simulink model "temperatureSource"  (R2016b)
settings: Solver=VariableStepAuto  StartTime=0.0  StopTime=10.0  RelTol=1e-3
libraries: fl_lib x4, nesl_utility x3
settings Model: Creator=Taeke  LastModifiedBy=Taeke

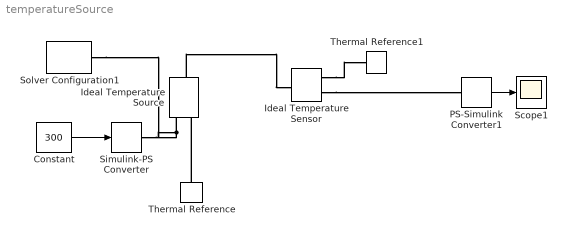
== system temperatureSource ==
  Constant : Constant  Value=300
  Ideal Temperature Sensor : fl_lib/Thermal/Thermal Sensors/Ideal Temperature Sensor
  Ideal Temperature Source : fl_lib/Thermal/Thermal Sources/Ideal Temperature Source
  PS-Simulink Converter1 : nesl_utility/PS-Simulink Converter  PhysicalDomain=network_engine_domain  SubClassName=ps_output  LeftPortType=input  RightPortType=output  PseudoPeriodic=off  Frequencies=[]  Unit=1  AffineConversion=off
  Scope1 : Scope
  Simulink-PS Converter : nesl_utility/Simulink-PS Converter  PhysicalDomain=network_engine_domain  SubClassName=ps_input  LeftPortType=input  RightPortType=output  PseudoPeriodic=off  Frequencies=[]  NoiseDistribution=none  NoiseParameters=[]  Unit=1  AffineConversion=off  InputFiltering=off  SimscapeFilterOrder=1  InputFilterTimeConstant=0.001  UdotUserProvided=1
  Solver Configuration1 : nesl_utility/Solver Configuration  PhysicalDomain=network_engine_domain  SubClassName=solver  LeftPortType=input  RightPortType=generic  Accelerate=off  Tones=[]  Harmonics=[]  SimulateNoise=off  Profile=off  UseLocalSampling=off  EnableSwitchedLinearOptims=on  FrequencyDomain=off  UseCCode=off  RelTol=0.001  AbsTol=1e-06  MinStep=1e-09  ToWorkspace=off  RevertToSquareIcSolve=off  NumHomotopyIterations=100  PhasorMode=off  PhasorModeNumHarmonics=1  OverrideAbsTol=off  DoDC=off  ResidualTolerance=1e-09  UseLocalSolver=off  LocalSolverChoice=NE_BACKWARD_EULER_ADVANCER  LocalSolverSampleTime=0.001  DoFixedCost=off  MaxNonlinIter=3  MaxModeIter=2  LinearAlgebra=Sparse  DelaysMemoryBudget=1024  AutomaticFiltering=on  FilteringTimeConstant=0.001
  Thermal Reference : fl_lib/Thermal/Thermal Elements/Thermal Reference
  Thermal Reference1 : fl_lib/Thermal/Thermal Elements/Thermal Reference
  wires:
  Constant/1 -> Simulink-PS Converter/1
  PS-Simulink Converter1/1 -> Scope1/1
  connections:
  Ideal Temperature Source/RConn1 -- Simulink-PS Converter/RConn1 -- Solver Configuration1/RConn1
  Ideal Temperature Sensor/RConn2 -- PS-Simulink Converter1/LConn1
  Ideal Temperature Source/LConn1 -- Ideal Temperature Sensor/LConn1
  Thermal Reference/LConn1 -- Ideal Temperature Source/RConn2
  Ideal Temperature Sensor/RConn1 -- Thermal Reference1/LConn1
